simulink model "RigidJoint_ConventionalSMC"  (R2019b)
settings: Solver=FixedStepAuto  StartTime=0.0  StopTime=10.0  FixedStep=0.002  RelTol=1e-3
libraries: robotcorelib x1
settings Model: Creator=USER  LastModifiedBy=USER
settings DebuggingCC: UnderSpecifiedDimensionMsg=warning

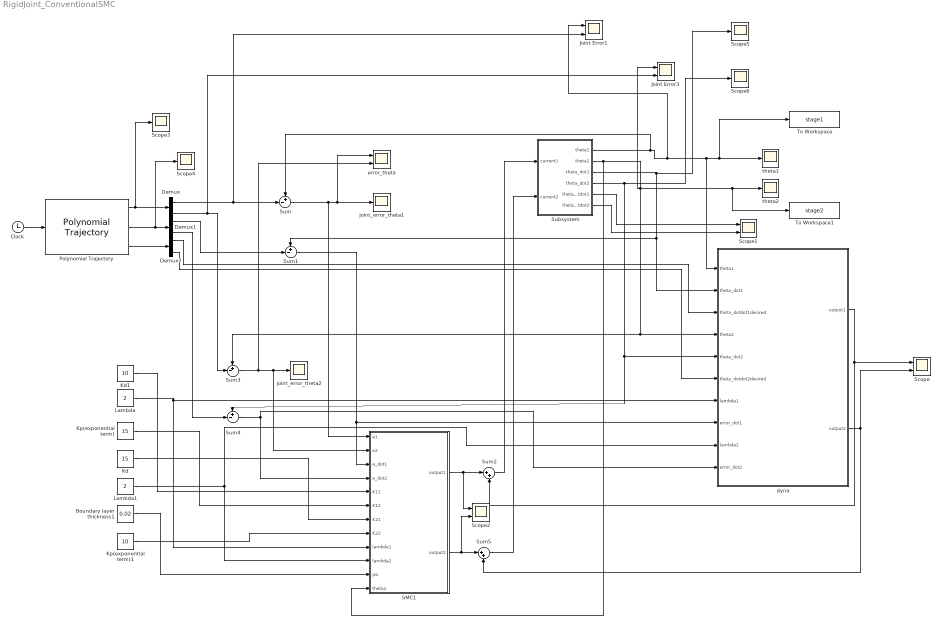
== system RigidJoint_ConventionalSMC ==
  Boundary layer thickness1 : Constant  Value=0.02
  Clock : Clock
  Demux : Demux  Outputs=2
  Demux1 : Demux  Outputs=2
  Demux2 : Demux  Outputs=2
  Joint Error1 : Scope  NumInputPorts=2
  Joint Error3 : Scope  NumInputPorts=2
  Kd : Constant  Value=15
  Kd1 : Constant  Value=10
  Kp(exponential term) : Constant  Value=15
  Kp(exponential term)1 : Constant  Value=10
  Lambda : Constant  Value=2
  Lambda1 : Constant  Value=2
  Polynomial Trajectory : robotcorelib/Polynomial Trajectory  WaypointSource=Internal  Waypoints=[ 0, pi/2; 0, pi/4]  TimePoints=[ 0, 5]  TimeInterval=[ 1, 4 ]  Method=Cubic Polynomial  ParameterSource=Internal  VelocityBoundaryCondition=zeros( 2, 2 )  AccelerationBoundaryCondition=zeros( 2, 5 )  SimulateUsing=Interpreted execution
      settings: SourceProductName=Robotics System Toolbox  SourceProductBaseCode=RO
  SMC1 : MATLAB Function  TreatAsAtomicUnit=on
  Scope : Scope  NumInputPorts=2
  Scope1 : Scope  NumInputPorts=2
  Scope2 : Scope  NumInputPorts=2
  Scope{3..6} (4 alike) : Scope
  Subsystem : Subsystem
  Sum{,1,3..4} (4 alike) : Sum  Inputs=+-|
  Sum2 : Sum  Inputs=|++
  Sum5 : Sum  Inputs=|++
  To Workspace : ToWorkspace  VariableName=stage1  SaveFormat=Timeseries  SampleTime=-1
  To Workspace1 : ToWorkspace  VariableName=stage2  SaveFormat=Timeseries  SampleTime=-1
  dyna : MATLAB Function  TreatAsAtomicUnit=on
  error_theta : Scope  NumInputPorts=2
  joint_error_theta1 : Scope
  joint_error_theta2 : Scope
  theta1 : Scope
  theta2 : Scope
  wires:
  Subsystem/1(theta1) -> Joint Error1/1, dyna/1(theta1), To Workspace/1, theta1/1, Sum/1
  Sum5/1 -> Subsystem/2("current2 ")
  Sum2/1 -> Subsystem/1(current1)
  SMC1/1(output1) -> Scope2/1, Sum2/1
  Subsystem/2(theta2) -> Joint Error3/1, To Workspace1/1, theta2/1, Sum3/1, dyna/4(theta2), SMC1/12(theta2)
  Demux1/1 -> Sum1/2
  Subsystem/6(theta_dotdot2) -> Scope1/2
  Sum1/1 -> SMC1/3(e_dot1), dyna/8(error_dot1)
  Subsystem/3(theta_dot1) -> Scope5/1, dyna/2(theta_dot1), Sum1/1
  Sum4/1 -> dyna/10(error_dot2), SMC1/4(e_dot2)
  Lambda/1 -> SMC1/9(lambda1), dyna/7(lambda1)
  Demux/2 -> Joint Error3/2, Sum3/2
  dyna/1(output1) -> Scope/1, Sum2/2
  Subsystem/4(theta_dot2) -> Scope6/1, Sum4/1, dyna/5(theta_dot2)
  dyna/2(output2) -> Scope/2, Sum5/2
  Sum/1 -> SMC1/1(e1), joint_error_theta1/1, error_theta/1
  Demux1/2 -> Sum4/2
  Sum3/1 -> SMC1/2(e2), joint_error_theta2/1, error_theta/2
  Lambda1/1 -> SMC1/10(lambda2), dyna/9(lambda2)
  Demux/1 -> Joint Error1/2, Sum/2
  Subsystem/5(theta_dotdot1) -> Scope1/1
  Polynomial Trajectory/1 -> Scope3/1, Demux/1
  Clock/1 -> Polynomial Trajectory/1
  Demux2/1 -> dyna/3(theta_dotdot1desired)
  Polynomial Trajectory/3 -> Demux2/1
  Demux2/2 -> dyna/6(theta_dotdot2desired)
  SMC1/2(output2) -> Scope2/2, Sum5/1
  Kd1/1 -> SMC1/5(K11)
  Kp(exponential term)1/1 -> SMC1/8(K22)
  Boundary layer thickness1/1 -> SMC1/11(psi)
  Kp(exponential term)/1 -> SMC1/6(K12)
  Kd/1 -> SMC1/7(K21)
  Polynomial Trajectory/2 -> Scope4/1, Demux1/1

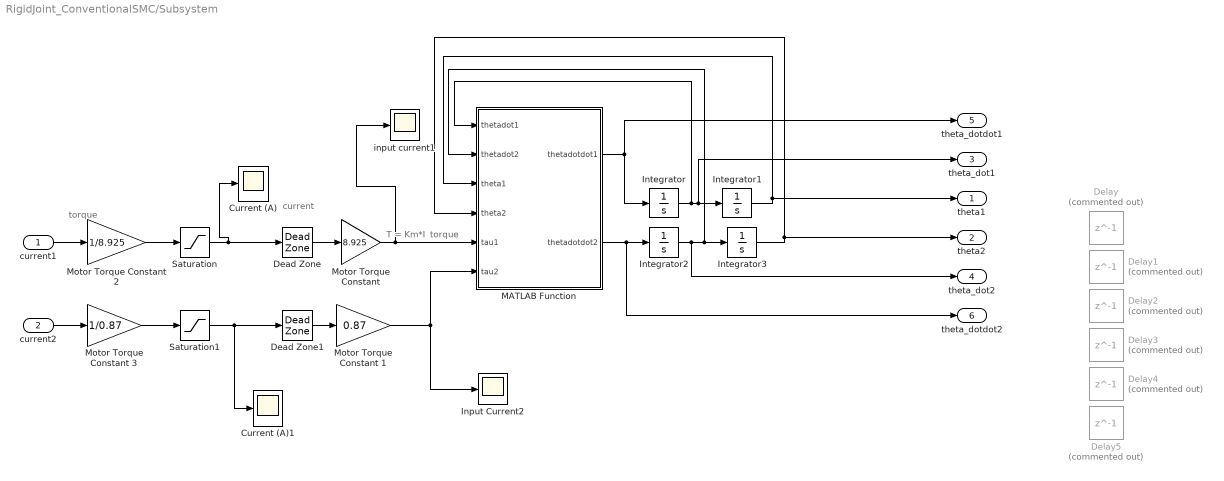
== system RigidJoint_ConventionalSMC/Subsystem ==
  note: current
  note: torque
  note: T = Km*I
  note: torque
  current1 : Inport
  "current2 " : Inport  Port=2
  Current (A) : Scope
  Current (A)1 : Scope
  Dead Zone : DeadZone  LowerValue=-0.15  UpperValue=0.15  SaturateOnIntegerOverflow=on
  Dead Zone1 : DeadZone  LowerValue=-0.15  UpperValue=0.15  SaturateOnIntegerOverflow=on
  Delay{,1..5} (6 alike) : Delay  Commented=on  DelayLength=1  SampleTime=0.002
  Input Current2 : Scope
  Integrator{,1..3} (4 alike) : Integrator
  MATLAB Function : MATLAB Function  TreatAsAtomicUnit=on
  "Motor Torque Constant " : Gain  Gain=8.925
  Motor Torque Constant 1 : Gain  Gain=0.87
  Motor Torque Constant 2 : Gain  Gain=1/8.925
  Motor Torque Constant 3 : Gain  Gain=1/0.87
  Saturation : Saturate  UpperLimit=0.94  LowerLimit=-0.94
  Saturation1 : Saturate  UpperLimit=0.94  LowerLimit=-0.94
  input current1 : Scope
  theta1 : Outport
  theta2 : Outport  Port=2
  theta_dot1 : Outport  Port=3
  theta_dot2 : Outport  Port=4
  theta_dotdot1 : Outport  Port=5
  theta_dotdot2 : Outport  Port=6
  wires:
  "Motor Torque Constant "/1 -> input current1/1, MATLAB Function/5(tau1)
  current1/1 -> Motor Torque Constant 2/1
  Motor Torque Constant 1/1 -> Input Current2/1, MATLAB Function/6(tau2)
  "current2 "/1 -> Motor Torque Constant 3/1
  MATLAB Function/1(thetadotdot1) -> theta_dotdot1/1, Integrator/1
  Integrator/1 -> MATLAB Function/1(thetadot1), theta_dot1/1, Integrator1/1
  Integrator1/1 -> theta1/1, MATLAB Function/3(theta1)
  Integrator3/1 -> theta2/1, MATLAB Function/4(theta2)
  Integrator2/1 -> theta_dot2/1, MATLAB Function/2(thetadot2), Integrator3/1
  MATLAB Function/2(thetadotdot2) -> theta_dotdot2/1, Integrator2/1
  Saturation/1 -> Current (A)/1, Dead Zone/1
  Saturation1/1 -> Current (A)1/1, Dead Zone1/1
  Motor Torque Constant 3/1 -> Saturation1/1
  Motor Torque Constant 2/1 -> Saturation/1
  Dead Zone/1 -> "Motor Torque Constant "/1
  Dead Zone1/1 -> Motor Torque Constant 1/1

== matlab function RigidJoint_ConventionalSMC/dyna ==
  data: theta1 input; output1 output; theta_dot1 input; theta_dotdot1desired input; theta2 input; theta_dot2 input; theta_dotdot2desired input; lambda1 input; error_dot1 input; lambda2 input; error_dot2 input; output2 output
function [output1, output2] = dyna(theta1, theta_dot1, theta_dotdot1desired, theta2, theta_dot2, theta_dotdot2desired, lambda1, error_dot1, lambda2, error_dot2)

m1 =  1.51 ; 
m2 = 0.87326;
L1 = 0.343;
L2 = 0.267;
Lc1 = 0.1590;
Lc2 = 0.0550;
I1 = 0.0392;
I2 = 0.0081;
B1 = 0.070364;
B2 = 0.028211;

% m1 = 0.5; 
% m2 = 1;
% L1 = 0.343;
% L2 = 0.267;
% Lc1 = 0.2;
% Lc2 = 0.25;
% I1 = 0.01;
% I2 = 0.01;
% B1 = 0.070364;
% B2 = 0.028211;
    
output1 = (theta_dotdot2desired - error_dot2*lambda2)*(m2*Lc2^2 + L1*m2*cos(theta2)*Lc2 + I2) - theta_dot2*(L1*Lc2*theta_dot1*m2*sin(theta2) + L1*Lc2*theta_dot2*m2*sin(theta2)) + B1*theta_dot1 + (theta_dotdot1desired - error_dot1*lambda1)*(I1 + I2 + m2*(L1^2 + 2*cos(theta2)*L1*Lc2 + Lc2^2) + Lc1^2*m1) - L1*Lc2*theta_dot1*theta_dot2*m2*sin(theta2);
output2 = L1*Lc2*m2*sin(theta2)*theta_dot1^2 + (theta_dotdot2desired - error_dot2*lambda2)*(m2*Lc2^2 + I2) + (theta_dotdot1desired - error_dot1*lambda1)*(m2*Lc2^2 + L1*m2*cos(theta2)*Lc2 + I2) + B2*theta_dot2;

end

== matlab function RigidJoint_ConventionalSMC/Subsystem/MATLAB Function ==
  data: thetadot1 input; thetadotdot1 output; thetadot2 input; theta1 input; theta2 input; tau1 input; thetadotdot2 output; tau2 input
function [thetadotdot1,thetadotdot2] = fcn(thetadot1,thetadot2,theta1,theta2,tau1,tau2)
%y is thetadotdot
tau = [tau1;tau2];
%Veltman Thesis Values
% m1 = 0.5; 
% m2 = 1;
% L1 = 0.343;
% L2 = 0.267;
% Lc1 = 0.2;
% Lc2 = 0.25;
% I1 = 0.01;
% I2 = 0.01;
% B1 = 0.070364;
% B2 = 0.028211;

%Electrical School values
% m1 =  1.51 ; 
% m2 = 0.87326;
% L1 = 0.343;
% L2 = 0.267;
% Lc1 = 0.1590;
% Lc2 = 0.0550;
% I1 = 0.0392;
% I2 = 0.0081;
% B1 = 0.070364;
% B2 = 0.028211;

%Robustnes Test
m1 =  2.0; 
m2 = 1.0;
L1 = 0.343;
L2 = 0.267;
Lc1 = 0.1590;
Lc2 = 0.0550;
I1 = 0.0392;
I2 = 0.0081;
B1 = 0.070364;
B2 = 0.028211;

M11 = I2+I1+m2*((L1^2)+(Lc2^2)+2*L1*Lc2*cos(theta2))+m1*(Lc1^2);
M12 = I2+m2*(Lc2^2)+L1*Lc2*m2*cos(theta2);
M21 = M12;
M22 = I2+m2*(Lc2^2);

M = [M11 M12;
     M21 M22];
 
C11 = -m2*L1*Lc2*sin(theta2)*thetadot2;
C12 = -m2*L1*Lc2*sin(theta2)*thetadot2-m2*L1*Lc2*sin(theta2)*thetadot1;
C21 = m2*L1*Lc2*sin(theta2)*thetadot1;
C22 = 0;

C = [C11 C12;
     C21 C22];

C1 = C*[thetadot1;thetadot2];
 
fv = [B1 0;0 B2]*[thetadot1;thetadot2];

thetadotdot = inv(M)*(tau-C1-fv);
thetadotdot1 = thetadotdot(1);
thetadotdot2 = thetadotdot(2);

== matlab function RigidJoint_ConventionalSMC/SMC1 ==
  data: e1 input; output1 output; e2 input; e_dot1 input; e_dot2 input; K11 input; K12 input; K21 input; K22 input; lambda1 input; lambda2 input; psi input; output2 output; theta2 input
function [output1, output2] = smc(e1, e2, e_dot1, e_dot2, K11, K12, K21, K22, lambda1, lambda2, psi, theta2)
    s1 = lambda1 * e1 + e_dot1;
    s2 = lambda2 * e2 + e_dot2;
         
    m1 =  1.51 ; 
    m2 = 0.87326;
    L1 = 0.343;
    L2 = 0.267;
    Lc1 = 0.1590;
    Lc2 = 0.0550;
    I1 = 0.0392;
    I2 = 0.0081;
    B1 = 0.070364;
    B2 = 0.028211;
    
    if (abs(s1) > psi)    
        sat_s1 = sign(s1);
    else
        sat_s1 = s1/psi;
    end
    
    if (abs(s2) > psi)    
        sat_s2 = sign(s2);
    else
        sat_s2 = s2/psi;
    end
    
%     output = (-Kd * sat_s - Kp*s)/(m2*Lc2^2 + I2);
    output1 = (-K21 * sat_s2 - K22*s2)*(m2*Lc2^2 + L1*m2*cos(theta2)*Lc2 + I2) + (-K11 * sat_s1 - K12*s1)*(I1 + I2 + m2*(L1^2 + 2*cos(theta2)*L1*Lc2 + Lc2^2) + Lc1^2*m1);
    output2 = (-K11 * sat_s1 - K12*s1)*(m2*Lc2^2 + L1*m2*cos(theta2)*Lc2 + I2) + (-K21 * sat_s2 - K22*s2)*(m2*Lc2^2 + I2);
end
